simulink model "smd_1202_sl"  (R2015b)
settings: Solver=ode1  SolverMode=SingleTasking  StartTime=0.0  StopTime=Inf  FixedStep=0.0001  RelTol=1e-3
PostLoadFcn:
  | , if any(exist('dsrtsu_mdlpostloadfcn', 'file') == [2, 3, 6]), try dsrtsu_mdlpostloadfcn('Execute', bdroot); catch fprintf('Error in PostLoadFcn (dsrtsu_mdlpostloadfcn) for model "%s":\n %s\n', bdroot, lasterr); end, end,
settings Model: RTICANMMDATA=struct('GeneralSetupData',struct('modelroot',['L:\New folder\REC_Maroje\Demo1\RTI\Demos\Model\GettingStarted\DS1202'],'generalsettings',struct('filesettings',struct('destfolder',struct('Name','RTICANMM_FILES','Check',1),'buildfolder',struct('Name','.','Check',1),'AbsDestfolder',struct('Name',['L:\New folder\REC_Maroje\Demo1\RTI\Demos\Model\GettingStarted\DS1202\RTICANMM_FILES']),'AbsBuildfolder',struct('Name',['L:\New folder\REC_Maroje\Demo1\RTI\Demos\Model\GettingStarted\DS1202']))),'options',struct('addpaths',1,'rmpaths',1,'addtrcexclusion',logical(1),'cannavigator',struct('checkmonitoring',0),'show_usrtrc',0,'use_usrtrc',0),'advanced',struct('options',ones(1,100)),'MPSetup',{{}},'modelname','smd_1202_sl','block','smd_1202_sl'))  RTILINMMDATA=struct('GeneralSetupData',[])  DSRTSU_INTERNAL_RTI_VER=500  DSRTSU_INTERNAL_RTI_TYPE=rti1202  DSRTSU_INTERNAL_RTIFLEXRAYCONFIG=110  DSRTSU_INTERNAL_RTIFPGA=90  ModifiedByFormat=dSPACE GmbH  ExtModeTrigMode=oneshot  ExtModeArmWhenConnect=off  ExtModeAutoUpdateStatusClock=off  Creator=dSPACE GmbH  LastModifiedBy=dSPACE GmbH
settings DataIOCC: SaveFormat=Array  SignalLoggingSaveFormat=ModelDataLogs
settings OptimizationCC: BlockReduction=off  ConditionallyExecuteInputs=off  OptimizeBlockIOStorage=off  BufferReuse=off  GlobalBufferReuse=off  ExpressionFolding=off  ExpressionDepthLimit=2147483647  LocalBlockOutputs=off  InitFltsAndDblsToZero=on
settings DebuggingCC: SaveWithParameterizedLinksMsg=none  UnderspecifiedInitializationDetection=Classic  MergeDetectMultiDrivingBlocksExec=none  SignalResolutionControl=TryResolveAllWithWarning  SolverPrmCheckMsg=warning  MultiTaskDSMMsg=warning  MultiTaskCondExecSysMsg=none  MultiTaskRateTransMsg=warning  TasksWithSamePriorityMsg=none  FcnCallInpInsideContextMsg=UseLocalSettings  StateNameClashWarn=warning
settings HardwareCC: ProdBitPerPointer=32  ProdLargestAtomicInteger=Integer  ProdEndianess=BigEndian  ProdWordSize=32  ProdHWDeviceType=Custom Processor->Custom  TargetIntDivRoundTo=Zero  TargetEndianess=BigEndian  TargetHWDeviceType=Custom Processor->Custom
settings RTWCC: SystemTargetFile=rti1202.tlc  MakeCommand=make_rti  TemplateMakefile=rti1202.tmf  Description=dSPACE DS1202 Hardware Platform  RTWVerbose=off
settings STFCustomTargetCC: ParMdlRefBuildCompliant=on  ConcurrentExecutionCompliant=off  GeneratePreprocessorConditionals=Use local settings  CPPClassGenCompliant=off  GRTInterface=off  SystemTargetFile=rti1202.tlc
settings GRTTargetCC: CompOptLevelCompliant=off  ConcurrentExecutionCompliant=off  CombineOutputUpdateFcns=off  MatFileLogging=off  CPPClassGenCompliant=off  UseToolchainInfoCompliant=off  ExtModeMexFile=noextcomm
settings ConfigComp: CovModelRefEnable=Off  CovSFcnEnable=off

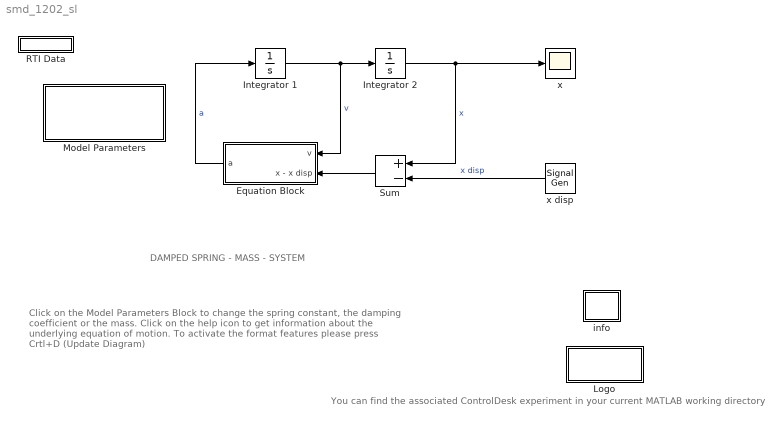
== system smd_1202_sl ==
  note: DAMPED SPRING - MASS - SYSTEM
  note: Click on the Model Parameters Block to change the spring constant,
      | the damping coefficient or the mass.
      | Click on the help icon to get information about the underlying equation
      | of motion.
      |
      | To activate the format features please
      | press Crtl+D (Update Diagram)
  note: You can find the associated ControlDesk experiment in your current MATLAB working directory
  Equation Block : Subsystem
  Integrator 1 : Integrator
  Integrator 2 : Integrator
  Logo : Subsystem  mask(dSPACE){EmptyParameter=[]}
      mask prompts: EmptyParameter "Mask Parameter 1:"
      settings: OpenFcn=;
      mask Display: image(imread('rti_mdl_dslogo.tif'));
  Model Parameters : Subsystem  mask{C=20000, d=16, m=0.04}
      mask prompts: C "Spring constant : C"; d "Damping coefficient : d"; m "Mass : m"
      mask Display: fprintf('Spring constant : C\nDamping coefficient : d\nMass : m')
  RTI Data : Subsystem  Tag=struct('RTIDataServer',struct('RTIDataServerVs','2','RTIModelDescription','struct(''main'',''smd_1202_sl'',''sub'','''',''isMp'',0)'))  LoadFcn="if exist('rtidc'), try,  rtidc('DataHostBlockClbLoad', gcbh); catch, disp(['Warning: ''LoadFcn'' for RTI Data block failed: ' lasterr]); end, end,"  mask(RTI_DATA_HOST){}
      mask help:
      | RTI Data Block.
      | This block is used by RTI to store internal model-dependent data.
      | Please keep this block on the root level of the model. Deleting this block will result in data loss.
      |
      | NEVER DELETE OR COPY THIS BLOCK!
      settings: CopyFcn="if exist('rtidc'), try,  rtidc('DataHostBlockClbCopy', gcbh); catch, disp(['Warning: ''CopyFcn'' for RTI Data block failed: ' lasterr]); end, end,"  DeleteFcn="if exist('rtidc'), try,  rtidc('DataHostBlockClbDelete', gcbh); catch, disp(['Warning: ''DeleteFcn'' for RTI Data block failed: ' lasterr]); end, end,"  ModelCloseFcn="if exist('rtidc'), try,  rtidc('DataHostBlockClbModelClose', gcbh); catch, disp(['Warning: ''ModelCloseFcn'' for RTI Data block failed: ' lasterr]); end, end,"  PreSaveFcn="if exist('rtidc'), try,  rtidc('DataHostBlockClbPreSave', gcbh); catch, disp(['Warning: ''PreSaveFcn'' for RTI Data block failed: ' lasterr]); end, end,"  PostSaveFcn="if exist('rtidc'), try,  rtidc('DataHostBlockClbPostSave', gcbh); catch, disp(['Warning: ''PostSaveFcn'' for RTI Data block failed: ' lasterr]); end, end,"  NameChangeFcn="if exist('rtidc'), try,  rtidc('DataHostBlockClbNameChange', gcbh); catch, disp(['Warning: ''NameChangeFcn'' for RTI Data block failed: ' lasterr]); end, end,"
      mask Help:
      | RTI Data Block.
      | This block is used by RTI to store internal model-dependent data.
      | Please keep this block on the root level of the model. Deleting this block will result in data loss.
      | 
      | NEVER DELETE OR COPY THIS BLOCK!
      mask Display:
      | text(0.5, 0.5, 'RTI Data', 'HorizontalAlignment', 'center');
      | plot([1 0]);
  Sum : Sum  Inputs=+-  SaturateOnIntegerOverflow=on  InputSameDT=on  OutDataTypeStr=Inherit: Same as first input
  info : Subsystem
      mask Display: disp('?')
  x : Scope
  x disp : SignalGenerator  WaveForm=square  Amplitude=0.5  Frequency=50
  wires:
  Integrator 1/1 -> Integrator 2/1, Equation Block/1(v)  "v"
  Sum/1 -> Equation Block/2(x - x disp)
  Equation Block/1(a) -> Integrator 1/1  "a"
  Integrator 2/1 -> Sum/1, x/1  "x"
  x disp/1 -> Sum/2  "x disp"

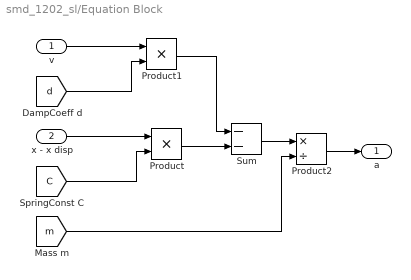
== system smd_1202_sl/Equation Block ==
  v : Inport
  x - x disp : Inport  Port=2
  Product : Product  SaturateOnIntegerOverflow=on  InputSameDT=on  OutDataTypeStr=Inherit: Same as first input
  Product1 : Product  SaturateOnIntegerOverflow=on  InputSameDT=on  OutDataTypeStr=Inherit: Same as first input
  Product2 : Product  Inputs=*/  SaturateOnIntegerOverflow=on  InputSameDT=on  OutDataTypeStr=Inherit: Same as first input
  Sum : Sum  Inputs=--  SaturateOnIntegerOverflow=on  InputSameDT=on  OutDataTypeStr=Inherit: Same as first input
  a : Outport
  wires:
  x - x disp/1 -> Product/1
  [C] -> Product/2
  v/1 -> Product1/1
  [d] -> Product1/2
  Product1/1 -> Sum/1
  Product/1 -> Sum/2
  Sum/1 -> Product2/1
  [m] -> Product2/2
  Product2/1 -> a/1

== system smd_1202_sl/Logo ==
  note: $Revision: 1.4 $
  note: $Date: 2013/06/17 16:41:25MESZ $
  note: $RCSfile: smd_1007_sl.mdl $

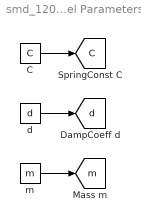
== system smd_1202_sl/Model Parameters ==
  C : Constant  Value=C
  d : Constant  Value=d
  m : Constant  Value=m
  tag scope: C=global, d=global, m=global
  wires:
  C/1 -> [C]
  d/1 -> [d]
  m/1 -> [m]

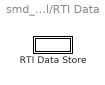
== system smd_1202_sl/RTI Data ==
  RTI Data Store : Subsystem  Tag="struct('private',struct('version',struct('dsVer',uint32(2)),'access',struct('modified',['03-Feb-2017 15:09:05'],'type','Model','isPerm',1)),'public',struct('main',struct('data',[]),'sub',struct('name',{{'smd_1202_sl'}},'data',{{struct('TH',struct('thTaskInfo',struct('taskType',{'TIMER','HWINT','TMRINT','SWINT','GLINT'},'tasksNumOf',{1,0,0,0,0},'srcIds',{{'TIMERA'},{},{},{},{}},'taskNames',{{['Timer Task 1']},{},{},{},{}})),'th_tc',struct('dataType','TASK','taskGroupId','','taskGroupList',{{}},'taskSchedulingPolicy','FCFS','taskType','TIMER','blkh',-1,'srcId','TIMERA','srcSgnName',['Timer A interrupt'],'srcCpuName','','taskName',['Timer Task 1  [0.0001] s'],'taskNameDisplayExt','','smplTime',0.0001,'smplTimeOffs',0,'hasFixedPriority',0,'priority',1,'hasFixedOvc',0,'ovcType',1,'ovcMax',1),'tc_th',struct('dataType','TASK','taskGroupId','','taskGroupList',{{}},'taskSchedulingPolicy','FCFS','taskType','TIMER','blkh',-1,'srcId','TIMERA','srcSgnName',['Timer A interrupt'],'srcCpuName','','taskName',['Timer Task 1  [0.0001] s'],'taskNameDisplayExt','','smplTime',0.0001,'smplTimeOffs',0,'hasFixedPriority',0,'priority',1,'hasFixedOvc',0,'ovcType',1,'ovcMax',1))}})))"  mask(RTI_DATA_STORE){}
      mask help:
      | RTI Data Store Block. This block is used by RTI to store internal model dependent data. Deleting this block will result in data loss.
      |
      | NEVER DELETE, COPY, OR MODIFY THIS BLOCK!
      mask Help:
      | RTI Data Store Block. This block is used by RTI to store internal model dependent data. Deleting this block will result in data loss.
      | 
      | NEVER DELETE, COPY, OR MODIFY THIS BLOCK!
      mask Display: text(0.5, 0.5, ' ', 'HorizontalAlignment', 'center');

== system smd_1202_sl/info ==
  note: a
      | d
      | m
      | v
      | C
      | x
      | x disp
      | f
      | t
      | u
  note: This demo example illustrates the behavior of a damped Spring-Mass-System.
      | After downloading the model to the DS1202, use ControlDesk NG to change the model para-
      | meters and to view the results.
      |
      | The equation of motion for the center of the mass driven by an external force is:
      |
      | a   =  -  (d / m) * v  -  (C / m)*( x - x disp )
  note: : acceleration of mass
      | : damping coeffecient
      | : mass
      | : velocity of the mass
      | : spring constant
      | : position of mass
      | : excitation
      | : frequency
      | : time
      | : amplitude of excitation
  note: The output of the Integrator 1 is v and is multiplied with d / m in the equation
      | block.
      | The output of the Integrator 2 is x. It  is added to x disp, and the sum is multiplied with
      | C / m in the equation block.
      | The output of the signal  generator is the exciting displacement of the mass:  x disp.
      |
      | In the case of a sine-like excitation the driving force is:
      | F = x disp * C
      | x disp  = u * cos ( 2pi * f * t)
      | The solution of the equation of motion is:
      | x ( t ) = xo * cos (2pi * f * t - alpha)
      | a harmonic oscillation with the original frequency, an amplitude xo and a phase alpha,
      | both depending on the model parameters.
      |
      | In the case of a square-like excitation the driving force results from a single displacement
      | of u, twice in the period T = 1 / f :
      | F = u * C
      | The solution of the equation of motion is:
      | x ( t ) = xo * exp[ - (d / 2m)* t ] * cos ( omega * t )
      | an exponentially decreasing sine wave with the natural frequency:
      | omega = sqrt [ (C / m) - ( d^2 / 4 m^2) ]
  note: MODEL SMD_1202_SL
  note: [m/s^2]
      | [kg/s]
      | [kg]
      | [m/s]
      | [kg/s^2]
      | [m]
      | [m]
      | [Hz]
      | [s]
      | [m]
  note: .

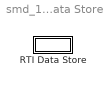
== system smd_1202_sl/RTI Data/RTI Data Store ==
  RTI Data Store : Subsystem  mask(RTI_DATA_STORE){}
      mask help:
      | RTI Data Store Block. This block is used by RTI to store internal model dependent data. Deleting this block will result in data loss.
      |
      | NEVER DELETE, COPY, OR MODIFY THIS BLOCK!
      mask Help:
      | RTI Data Store Block. This block is used by RTI to store internal model dependent data. Deleting this block will result in data loss.
      | 
      | NEVER DELETE, COPY, OR MODIFY THIS BLOCK!
      mask Display: text(0.5, 0.5, ' ', 'HorizontalAlignment', 'center');

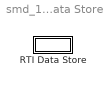
== system smd_1202_sl/RTI Data/RTI Data Store/RTI Data Store ==
  RTI Data Store : Subsystem  mask(RTI_DATA_STORE){}
      mask help:
      | RTI Data Store Block. This block is used by RTI to store internal model dependent data. Deleting this block will result in data loss.
      |
      | NEVER DELETE, COPY, OR MODIFY THIS BLOCK!
      mask Help:
      | RTI Data Store Block. This block is used by RTI to store internal model dependent data. Deleting this block will result in data loss.
      | 
      | NEVER DELETE, COPY, OR MODIFY THIS BLOCK!
      mask Display: text(0.5, 0.5, ' ', 'HorizontalAlignment', 'center');

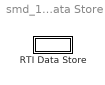
== system smd_1202_sl/RTI Data/RTI Data Store/RTI Data Store/RTI Data Store ==
  RTI Data Store : Subsystem  mask(RTI_DATA_STORE){}
      mask help:
      | RTI Data Store Block. This block is used by RTI to store internal model dependent data. Deleting this block will result in data loss.
      |
      | NEVER DELETE, COPY, OR MODIFY THIS BLOCK!
      mask Help:
      | RTI Data Store Block. This block is used by RTI to store internal model dependent data. Deleting this block will result in data loss.
      | 
      | NEVER DELETE, COPY, OR MODIFY THIS BLOCK!
      mask Display: text(0.5, 0.5, ' ', 'HorizontalAlignment', 'center');

== system smd_1202_sl/RTI Data/RTI Data Store/RTI Data Store/RTI Data Store/RTI Data Store ==
